simulink model "MPC_Ctr_2016b"  (Simulink 8.8)
settings: Solver=ode1  StartTime=0.0  StopTime=20  FixedStep=0.0001  RelTol=1e-3
values from neighbouring files (symbols this model uses):
  A_disc = sys_disc.A    [MPC.m]
  B_disc = sys_disc.B    [MPC.m]
  C_disc = sys_disc.C    [MPC.m]
  D_disc = sys_disc.D    [MPC.m]
  E = C'*Q_bar*M    [MPC_Matrices.m]
  H = C'*Q_bar*C+R_bar    [MPC_Matrices.m]
  Time_step = 0.03    [MPC.m]
undefined symbols (not defined in the file or in its folder): K
settings Model: Creator=gaoaidi  LastModifiedBy=15324
settings DataIOCC: LimitDataPoints=off  SaveFormat=Dataset  SignalLoggingSaveFormat=Dataset  ReturnWorkspaceOutputs=on
settings OptimizationCC: LifeSpan=auto
settings DebuggingCC: UnderspecifiedInitializationDetection=Simplified  MergeDetectMultiDrivingBlocksExec=error  FcnCallInpInsideContextMsg=error  StateNameClashWarn=none  SFUnexpectedBacktrackingDiag=error  SFNoUnconditionalDefaultTransitionDiag=error  SFExecutionAtInitializationDiag=warning
settings HardwareCC: ProdBitPerPointer=64  ProdBitPerSizeT=64  ProdBitPerPtrDiffT=64  ProdLargestAtomicFloat=Float  ProdIntDivRoundTo=Zero  ProdEndianess=LittleEndian  ProdWordSize=64  ProdHWDeviceType=Intel->x86-64 (Windows64)
settings ModelReferenceCC: PropagateSignalLabelsOutOfModel=on
settings SFSimCC: SimUseLocalCustomCode=on
settings RTWCC: RTWUseLocalCustomCode=on
settings GRTTargetCC: TargetLangStandard=C99 (ISO)  CombineOutputUpdateFcns=on  GRTInterface=off
settings ConfigComp: CovMetricSettings=dwe  CovSaveCumulativeToWorkspaceVar=off  CovSaveSingleToWorkspaceVar=off  CovExternalEMLEnable=on

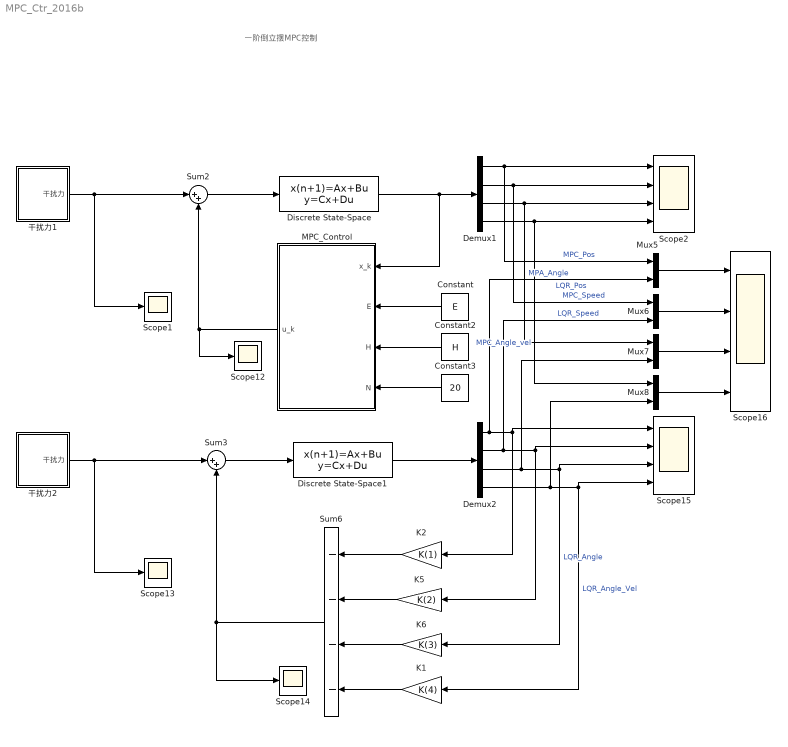
== system MPC_Ctr_2016b ==
  note: 一阶倒立摆MPC控制
  Constant : Constant  Value=E  VectorParams1D=off
  Constant2 : Constant  Value=H  VectorParams1D=off
  Constant3 : Constant  Value=20
  Demux1 : Demux
  Demux2 : Demux
  Discrete State-Space : DiscreteStateSpace  A=A_disc  B=B_disc  C=C_disc  D=D_disc  SampleTime=Time_step
  Discrete State-Space1 : DiscreteStateSpace  A=A_disc  B=B_disc  C=C_disc  D=D_disc  SampleTime=Time_step
  K1 : Gain  Gain=K(4)
  K2 : Gain  Gain=K(1)
  K5 : Gain  Gain=K(2)
  K6 : Gain  Gain=K(3)
  MPC_Control : MATLAB Function  TreatAsAtomicUnit=on
  Mux{5..8} (4 alike) : Mux  Inputs=2
  Scope{1,12..14} (4 alike) : Scope
  Scope15 : Scope  NumInputPorts=4
  Scope16 : Scope  NumInputPorts=4
  Scope2 : Scope  NumInputPorts=4
  Sum2 : Sum  Inputs=|++
  Sum3 : Sum  Inputs=|++
  Sum6 : Sum  Inputs=----
  干扰力1 : Subsystem  mask{Input=<empty>}
      mask prompts: Input "干扰力类型"
  干扰力2 : Subsystem  mask{Input=<empty>}
      mask prompts: Input "干扰力类型"
  wires:
  干扰力1/1(干扰力) -> Scope1/1, Sum2/1
  Demux1/4 -> Mux8/1, Scope2/4  "MPC_Angle_vel"
  Demux1/2 -> Scope2/2, Mux6/1  "MPC_Speed"
  Demux1/3 -> Mux7/1, Scope2/3  "MPA_Angle"
  Demux1/1 -> Scope2/1, Mux5/1  "MPC_Pos"
  Sum2/1 -> Discrete State-Space/1
  Discrete State-Space/1 -> MPC_Control/1(x_k), Demux1/1
  MPC_Control/1(u_k) -> Scope12/1, Sum2/2
  Constant/1 -> MPC_Control/2(E)
  Constant2/1 -> MPC_Control/3(H)
  Constant3/1 -> MPC_Control/4(N)
  干扰力2/1(干扰力) -> Scope13/1, Sum3/1
  Discrete State-Space1/1 -> Demux2/1
  Sum3/1 -> Discrete State-Space1/1
  Demux2/1 -> Scope15/1, K2/1, Mux5/2  "LQR_Pos"
  K1/1 -> Sum6/4
  K2/1 -> Sum6/1
  K6/1 -> Sum6/3
  Demux2/3 -> Mux7/2, K6/1, Scope15/3  "LQR_Angle"
  Demux2/2 -> K5/1, Scope15/2, Mux6/2  "LQR_Speed"
  Sum6/1 -> Scope14/1, Sum3/2
  K5/1 -> Sum6/2
  Demux2/4 -> Mux8/2, K1/1, Scope15/4  "LQR_Angle_Vel"
  Mux5/1 -> Scope16/1
  Mux6/1 -> Scope16/2
  Mux7/1 -> Scope16/3
  Mux8/1 -> Scope16/4

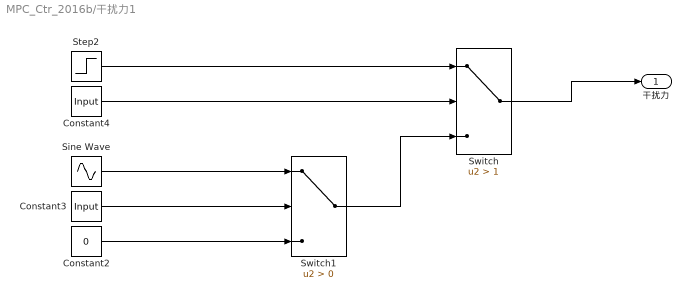
== system MPC_Ctr_2016b/干扰力1 ==
  Constant2 : Constant  Value=0
  Constant3 : Constant  Value=Input
  Constant4 : Constant  Value=Input
  Sine Wave : Sin  SampleTime=Time_step
  Step2 : Step  Before=20  After=0  SampleTime=Time_step
  Switch : Switch  Criteria=u2 > Threshold  Threshold=1
  Switch1 : Switch  Criteria=u2 > Threshold
  干扰力 : Outport
  wires:
  Constant4/1 -> Switch/2
  Constant2/1 -> Switch1/3
  Switch/1 -> 干扰力/1
  Constant3/1 -> Switch1/2
  Switch1/1 -> Switch/3
  Sine Wave/1 -> Switch1/1
  Step2/1 -> Switch/1

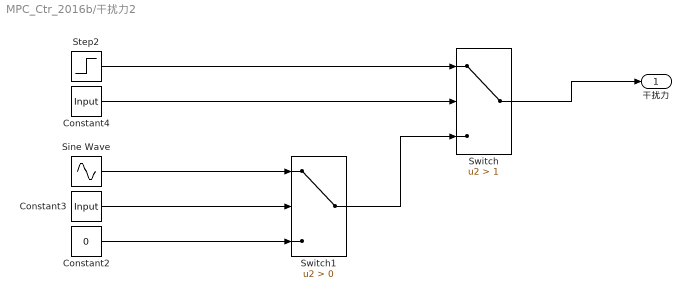
== system MPC_Ctr_2016b/干扰力2 ==
  Constant2 : Constant  Value=0
  Constant3 : Constant  Value=Input
  Constant4 : Constant  Value=Input
  Sine Wave : Sin  Amplitude=0.5  SampleTime=Time_step
  Step2 : Step  Before=20  After=0  SampleTime=Time_step
  Switch : Switch  Criteria=u2 > Threshold  Threshold=1
  Switch1 : Switch  Criteria=u2 > Threshold
  干扰力 : Outport
  wires:
  Constant4/1 -> Switch/2
  Constant2/1 -> Switch1/3
  Switch/1 -> 干扰力/1
  Constant3/1 -> Switch1/2
  Switch1/1 -> Switch/3
  Sine Wave/1 -> Switch1/1
  Step2/1 -> Switch/1

== matlab function MPC_Control ==
  data: x_k input double; u_k output double; E input double; H input double; N input double
function u_k = Prediction(x_k, E, H, N)  
    % 初始化输出  
    U_k = zeros(N*1, 1); % NP x 1  
    u_k = zeros(1, 1); % 指定 u_k 为固定大小 p x 1

    % 获取 H 矩阵的行列数
    [m, n] = size(H);

    % 根据 H 矩阵的列数定义初始向量 x0
    x0 = zeros(n, 1);
    % 使用quadprog函数求解优化问题  
    opts = optimoptions('quadprog','Algorithm','active-set');
    [U_k, ~, ~] = quadprog(H, E * x_k, [], [], [], [], [], [], x0, opts);
      
    % 取第一个结果  
    u_k = U_k(1, 1);  
end
